simulink library "Loudness"  (R2022b)
settings: Solver=VariableStepAuto  StartTime=0.0  StopTime=10.0  RelTol=1e-3
InitFcn:
  | Loudness_init;
values from neighbouring files (symbols this model uses):
  COMP = struct('zipCoef', COMP_zipCoef,      'LoudBPFNum', COMPBASS_Num, 'LoudBPFDenom', COMPBASS_Denom,      'LoudLPFNum', COMPMID_Num, 'LoudLPFDenom', COMPMID_Denom,      'LoudBPFFreq',COMPBASS_Fc,'LoudBPFQ',COMPBASS_Q,      'LoudLPFFreq',COMPMID_Fc,'LoudLPFQ',COMPMID_Q)    [Loudness_init.m]
undefined symbols (not defined in the file or in its folder): dfilt, LOUD_BASS_0DB_SCALE, LOUD_BASS_D1, LOUD_BASS_D2, sys_defs
libraries: TuneVar x38, RTC x16, dspobslib x5
(part 1 of 2)
settings Model: Creator=jb10849  LastModifiedBy=kl13806
settings SolverCC: AlgebraicLoopSolver=TrustRegion
settings DebuggingCC: UnconnectedInputMsg=warning  UnconnectedOutputMsg=warning  UnconnectedLineMsg=warning  SFMachineParentedDataDiag=warning  ArithmeticOperatorsInVariantConditions=warning
settings ModelReferenceCC: EnableRefExpFcnMdlSchedulingChecks=on
settings SFSimCC: SimUseLocalCustomCode=off  CustomCodeUndefinedFunction=UseInterfaceOnly
settings RTWCC: RTWUseLocalCustomCode=off  DLArmComputeVersion=19.05
settings CodeAppCC: StateflowObjectComments=on

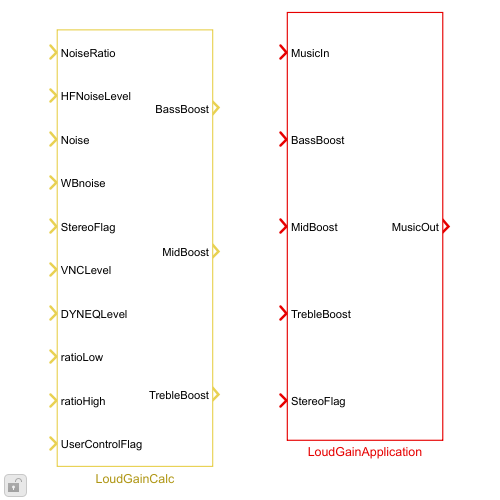
[thumbnail: Simulink's stored preview of the top-level diagram]
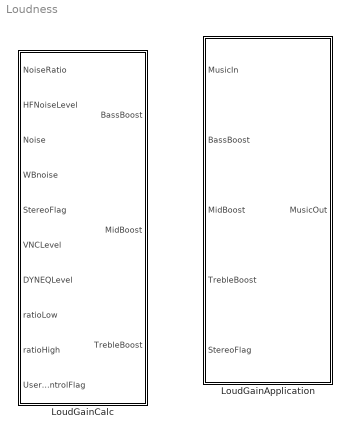
== system Loudness ==
  LoudGainApplication : Subsystem  mask(Loudness Gain Application){}
      mask help: Loudness gain application for Audio Pilot.
  LoudGainCalc : Subsystem  mask(Loudness Gain Calculation){}
      mask help: Loudness gain calculation for Audio Pilot.

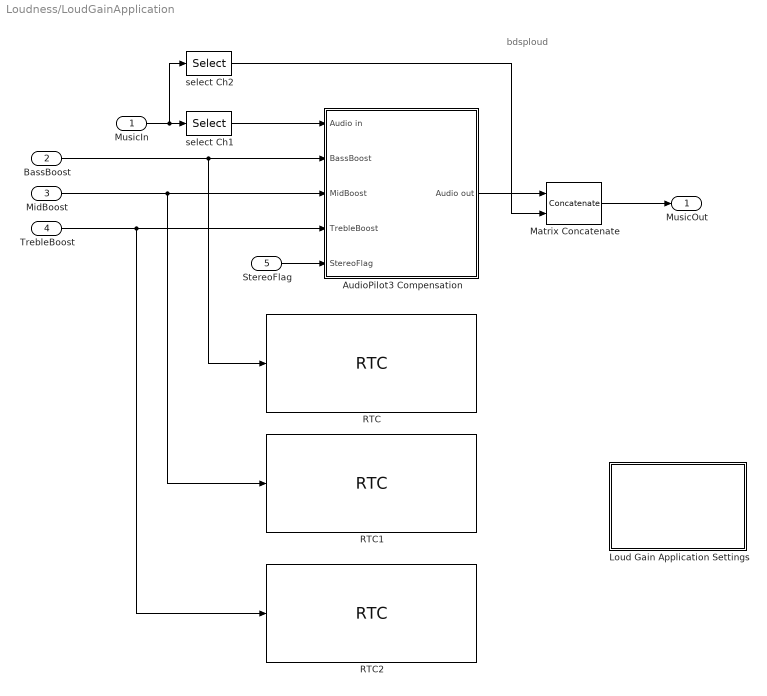
== system Loudness/LoudGainApplication ==
  note: bdsploud
  MusicIn : Inport
  BassBoost : Inport  Port=2
  MidBoost : Inport  Port=3
  TrebleBoost : Inport  Port=4
  StereoFlag : Inport  Port=5
  AudioPilot3 Compensation : Subsystem
  Loud Gain Application Settings : Subsystem
  Matrix Concatenate : Concatenate  Mode=Multidimensional array  ConcatenateDimension=2
  RTC : RTC/RTC  REQ_Priority=RTC_Mask.NormalPriority  RequestAtInit=off  EnableRequest=off  REQElemType1=single  REQElemWidth1=1  REQElemInitial1=[]  REQElemType2=uint32  REQElemWidth2=1  REQElemInitial2=[]  REQElemType3=uint32  REQElemWidth3=1  REQElemInitial3=[]  REQElemType4=uint32  REQElemWidth4=1  REQElemInitial4=[]  REQElemType5=uint32  REQElemWidth5=1  REQElemInitial5=[]  REQElemType6=uint32  REQElemWidth6=1  REQElemInitial6=[]  REQElemType7=uint32  REQElemWidth7=1  REQElemInitial7=[]  REQElemType8=uint32  REQElemWidth8=1  REQElemInitial8=[]  REQElemType9=uint32  REQElemWidth9=1  REQElemInitial9=[]  REQElemType10=uint32  REQElemWidth10=1  REQElemInitial10=[]  EnableResponse=on  EnableRSP_StatusIn=off  RSPElemName1=bassBoost  RSPElemType1=single  RSPElemWidth1=1  RSPElemType2=uint32  RSPElemWidth2=1  RSPElemType3=uint32  RSPElemWidth3=1  RSPElemType4=uint32  RSPElemWidth4=1  RSPElemType5=uint32  RSPElemWidth5=1  RSPElemType6=uint32  RSPElemWidth6=1  RSPElemType7=uint32  RSPElemWidth7=1  RSPElemType8=uint32  RSPElemWidth8=1  RSPElemType9=uint32  RSPElemWidth9=1  RSPElemType10=uint32  RSPElemWidth10=1  EnableNotification=off  EnableNTF_PrepTrig=off  NTFElemType1=uint32  NTFElemWidth1=1  NTFElemType2=uint32  NTFElemWidth2=1  NTFElemType3=uint32  NTFElemWidth3=1  NTFElemType4=uint32  NTFElemWidth4=1  NTFElemType5=uint32  NTFElemWidth5=1  NTFElemType6=uint32  NTFElemWidth6=1  NTFElemType7=uint32  NTFElemWidth7=1  NTFElemType8=uint32  NTFElemWidth8=1  NTFElemType9=uint32  NTFElemWidth9=1  NTFElemType10=uint32  NTFElemWidth10=1  MaskMessageName=getBassBoost
  RTC1 : RTC/RTC  REQ_Priority=RTC_Mask.NormalPriority  RequestAtInit=off  EnableRequest=off  REQElemType1=single  REQElemWidth1=1  REQElemInitial1=[]  REQElemType2=uint32  REQElemWidth2=1  REQElemInitial2=[]  REQElemType3=uint32  REQElemWidth3=1  REQElemInitial3=[]  REQElemType4=uint32  REQElemWidth4=1  REQElemInitial4=[]  REQElemType5=uint32  REQElemWidth5=1  REQElemInitial5=[]  REQElemType6=uint32  REQElemWidth6=1  REQElemInitial6=[]  REQElemType7=uint32  REQElemWidth7=1  REQElemInitial7=[]  REQElemType8=uint32  REQElemWidth8=1  REQElemInitial8=[]  REQElemType9=uint32  REQElemWidth9=1  REQElemInitial9=[]  REQElemType10=uint32  REQElemWidth10=1  REQElemInitial10=[]  EnableResponse=on  EnableRSP_StatusIn=off  RSPElemName1=midBoost  RSPElemType1=single  RSPElemWidth1=1  RSPElemType2=uint32  RSPElemWidth2=1  RSPElemType3=uint32  RSPElemWidth3=1  RSPElemType4=uint32  RSPElemWidth4=1  RSPElemType5=uint32  RSPElemWidth5=1  RSPElemType6=uint32  RSPElemWidth6=1  RSPElemType7=uint32  RSPElemWidth7=1  RSPElemType8=uint32  RSPElemWidth8=1  RSPElemType9=uint32  RSPElemWidth9=1  RSPElemType10=uint32  RSPElemWidth10=1  EnableNotification=off  EnableNTF_PrepTrig=off  NTFElemType1=uint32  NTFElemWidth1=1  NTFElemType2=uint32  NTFElemWidth2=1  NTFElemType3=uint32  NTFElemWidth3=1  NTFElemType4=uint32  NTFElemWidth4=1  NTFElemType5=uint32  NTFElemWidth5=1  NTFElemType6=uint32  NTFElemWidth6=1  NTFElemType7=uint32  NTFElemWidth7=1  NTFElemType8=uint32  NTFElemWidth8=1  NTFElemType9=uint32  NTFElemWidth9=1  NTFElemType10=uint32  NTFElemWidth10=1  MaskMessageName=getMidBoost
  RTC2 : RTC/RTC  REQ_Priority=RTC_Mask.NormalPriority  RequestAtInit=off  EnableRequest=off  REQElemType1=single  REQElemWidth1=1  REQElemInitial1=[]  REQElemType2=uint32  REQElemWidth2=1  REQElemInitial2=[]  REQElemType3=uint32  REQElemWidth3=1  REQElemInitial3=[]  REQElemType4=uint32  REQElemWidth4=1  REQElemInitial4=[]  REQElemType5=uint32  REQElemWidth5=1  REQElemInitial5=[]  REQElemType6=uint32  REQElemWidth6=1  REQElemInitial6=[]  REQElemType7=uint32  REQElemWidth7=1  REQElemInitial7=[]  REQElemType8=uint32  REQElemWidth8=1  REQElemInitial8=[]  REQElemType9=uint32  REQElemWidth9=1  REQElemInitial9=[]  REQElemType10=uint32  REQElemWidth10=1  REQElemInitial10=[]  EnableResponse=on  EnableRSP_StatusIn=off  RSPElemName1=trebleBoost  RSPElemType1=single  RSPElemWidth1=1  RSPElemType2=uint32  RSPElemWidth2=1  RSPElemType3=uint32  RSPElemWidth3=1  RSPElemType4=uint32  RSPElemWidth4=1  RSPElemType5=uint32  RSPElemWidth5=1  RSPElemType6=uint32  RSPElemWidth6=1  RSPElemType7=uint32  RSPElemWidth7=1  RSPElemType8=uint32  RSPElemWidth8=1  RSPElemType9=uint32  RSPElemWidth9=1  RSPElemType10=uint32  RSPElemWidth10=1  EnableNotification=off  EnableNTF_PrepTrig=off  NTFElemType1=uint32  NTFElemWidth1=1  NTFElemType2=uint32  NTFElemWidth2=1  NTFElemType3=uint32  NTFElemWidth3=1  NTFElemType4=uint32  NTFElemWidth4=1  NTFElemType5=uint32  NTFElemWidth5=1  NTFElemType6=uint32  NTFElemWidth6=1  NTFElemType7=uint32  NTFElemWidth7=1  NTFElemType8=uint32  NTFElemWidth8=1  NTFElemType9=uint32  NTFElemWidth9=1  NTFElemType10=uint32  NTFElemWidth10=1  MaskMessageName=getTrebleBoost
  select Ch1 : Selector  NumberOfDimensions=2  InputPortWidth=3  IndexOptions=Select all,Index vector (dialog)  Indices=[1 3],1:2  OutputSizes=1,1
  select Ch2 : Selector  NumberOfDimensions=2  InputPortWidth=3  IndexOptions=Select all,Index vector (dialog)  Indices=[1 3],3:6  OutputSizes=1,1
  MusicOut : Outport  VectorParamsAs1DForOutWhenUnconnected=off
  wires:
  MusicIn/1 -> select Ch2/1, select Ch1/1
  MidBoost/1 -> AudioPilot3 Compensation/3(MidBoost), RTC1/1
  TrebleBoost/1 -> AudioPilot3 Compensation/4(TrebleBoost), RTC2/1
  BassBoost/1 -> AudioPilot3 Compensation/2(BassBoost), RTC/1
  select Ch1/1 -> AudioPilot3 Compensation/1(Audio in)
  AudioPilot3 Compensation/1(Audio out) -> Matrix Concatenate/1
  Matrix Concatenate/1 -> MusicOut/1
  select Ch2/1 -> Matrix Concatenate/2
  StereoFlag/1 -> AudioPilot3 Compensation/5(StereoFlag)

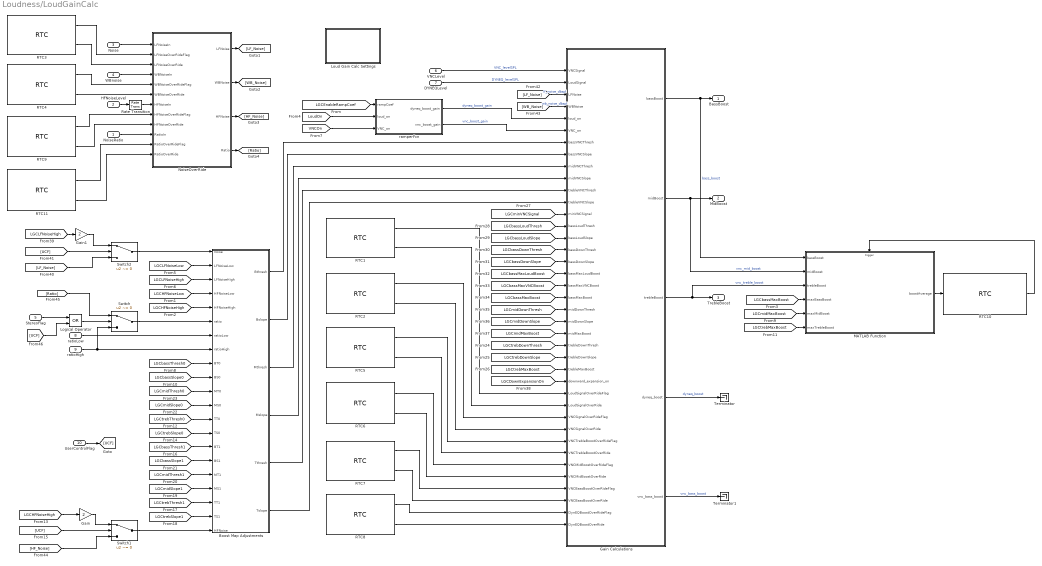
== system Loudness/LoudGainCalc ==
  NoiseRatio : Inport
  HFNoiseLevel : Inport  Port=2
  Noise : Inport  Port=3
  WBnoise : Inport  Port=4
  StereoFlag : Inport  Port=5
  VNCLevel : Inport  Port=6
  DYNEQLevel : Inport  Port=7
  ratioLow : Inport  Port=8
  ratioHigh : Inport  Port=9
  UserControlFlag : Inport  Port=10
  Boost Map Adjustments : MATLAB Function  TreatAsAtomicUnit=on
  Gain : Gain  Gain=2
  Gain Calculations : MATLAB Function  TreatAsAtomicUnit=on
  Gain1 : Gain  Gain=2
  Logical Operator : Logic  Operator=OR  AllPortsSameDT=off  OutDataTypeStr=boolean
  Loud Gain Calc Settings : Subsystem
  MATLAB Function : MATLAB Function  TreatAsAtomicUnit=on
  NoiseOverRide : MATLAB Function  TreatAsAtomicUnit=on
  RTC1 : RTC/RTC  REQ_Priority=RTC_Mask.NormalPriority  RequestAtInit=off  EnableRequest=off  REQElemName1=LoudSignalOverRideFlag  REQElemType1=uint32  REQElemWidth1=1  REQElemInitial1=[]  REQElemName2=LoudSignalOverRide  REQElemType2=single  REQElemWidth2=1  REQElemInitial2=[]  REQElemType3=uint32  REQElemWidth3=1  REQElemInitial3=[]  REQElemType4=uint32  REQElemWidth4=1  REQElemInitial4=[]  REQElemType5=uint32  REQElemWidth5=1  REQElemInitial5=[]  REQElemType6=uint32  REQElemWidth6=1  REQElemInitial6=[]  REQElemType7=uint32  REQElemWidth7=1  REQElemInitial7=[]  REQElemType8=uint32  REQElemWidth8=1  REQElemInitial8=[]  REQElemType9=uint32  REQElemWidth9=1  REQElemInitial9=[]  REQElemType10=uint32  REQElemWidth10=1  REQElemInitial10=[]  EnableResponse=off  EnableRSP_StatusIn=off  RSPElemType1=uint32  RSPElemWidth1=1  RSPElemType2=uint32  RSPElemWidth2=1  RSPElemType3=uint32  RSPElemWidth3=1  RSPElemType4=uint32  RSPElemWidth4=1  RSPElemType5=uint32  RSPElemWidth5=1  RSPElemType6=uint32  RSPElemWidth6=1  RSPElemType7=uint32  RSPElemWidth7=1  RSPElemType8=uint32  RSPElemWidth8=1  RSPElemType9=uint32  RSPElemWidth9=1  RSPElemType10=uint32  RSPElemWidth10=1  EnableNotification=off  EnableNTF_PrepTrig=off  NTFElemType1=uint32  NTFElemWidth1=1  NTFElemType2=uint32  NTFElemWidth2=1  NTFElemType3=uint32  NTFElemWidth3=1  NTFElemType4=uint32  NTFElemWidth4=1  NTFElemType5=uint32  NTFElemWidth5=1  NTFElemType6=uint32  NTFElemWidth6=1  NTFElemType7=uint32  NTFElemWidth7=1  NTFElemType8=uint32  NTFElemWidth8=1  NTFElemType9=uint32  NTFElemWidth9=1  NTFElemType10=uint32  NTFElemWidth10=1  MaskMessageName=setLoudSignalOverRide
  RTC10 : RTC/RTC  REQ_Priority=RTC_Mask.NormalPriority  RequestAtInit=off  EnableRequest=on  REQElemType1=uint32  REQElemWidth1=1  REQElemInitial1=[]  REQElemType2=uint32  REQElemWidth2=1  REQElemInitial2=[]  REQElemType3=uint32  REQElemWidth3=1  REQElemInitial3=[]  REQElemType4=uint32  REQElemWidth4=1  REQElemInitial4=[]  REQElemType5=uint32  REQElemWidth5=1  REQElemInitial5=[]  REQElemType6=uint32  REQElemWidth6=1  REQElemInitial6=[]  REQElemType7=uint32  REQElemWidth7=1  REQElemInitial7=[]  REQElemType8=uint32  REQElemWidth8=1  REQElemInitial8=[]  REQElemType9=uint32  REQElemWidth9=1  REQElemInitial9=[]  REQElemType10=uint32  REQElemWidth10=1  REQElemInitial10=[]  EnableResponse=on  EnableRSP_StatusIn=off  RSPElemName1=level  RSPElemType1=single  RSPElemWidth1=1  RSPElemType2=uint32  RSPElemWidth2=1  RSPElemType3=uint32  RSPElemWidth3=1  RSPElemType4=uint32  RSPElemWidth4=1  RSPElemType5=uint32  RSPElemWidth5=1  RSPElemType6=uint32  RSPElemWidth6=1  RSPElemType7=uint32  RSPElemWidth7=1  RSPElemType8=uint32  RSPElemWidth8=1  RSPElemType9=uint32  RSPElemWidth9=1  RSPElemType10=uint32  RSPElemWidth10=1  EnableNotification=off  EnableNTF_PrepTrig=off  NTFElemType1=uint32  NTFElemWidth1=1  NTFElemType2=uint32  NTFElemWidth2=1  NTFElemType3=uint32  NTFElemWidth3=1  NTFElemType4=uint32  NTFElemWidth4=1  NTFElemType5=uint32  NTFElemWidth5=1  NTFElemType6=uint32  NTFElemWidth6=1  NTFElemType7=uint32  NTFElemWidth7=1  NTFElemType8=uint32  NTFElemWidth8=1  NTFElemType9=uint32  NTFElemWidth9=1  NTFElemType10=uint32  NTFElemWidth10=1  MaskMessageName=getAverageAudioPilotBoostLevel
  RTC11 : RTC/RTC  REQ_Priority=RTC_Mask.NormalPriority  RequestAtInit=off  EnableRequest=off  REQElemName1=RatioOverRideFlag  REQElemType1=uint32  REQElemWidth1=1  REQElemInitial1=[]  REQElemName2=RatioOverRide  REQElemType2=single  REQElemWidth2=1  REQElemInitial2=[]  REQElemType3=uint32  REQElemWidth3=1  REQElemInitial3=[]  REQElemType4=uint32  REQElemWidth4=1  REQElemInitial4=[]  REQElemType5=uint32  REQElemWidth5=1  REQElemInitial5=[]  REQElemType6=uint32  REQElemWidth6=1  REQElemInitial6=[]  REQElemType7=uint32  REQElemWidth7=1  REQElemInitial7=[]  REQElemType8=uint32  REQElemWidth8=1  REQElemInitial8=[]  REQElemType9=uint32  REQElemWidth9=1  REQElemInitial9=[]  REQElemType10=uint32  REQElemWidth10=1  REQElemInitial10=[]  EnableResponse=off  EnableRSP_StatusIn=off  RSPElemType1=uint32  RSPElemWidth1=1  RSPElemType2=uint32  RSPElemWidth2=1  RSPElemType3=uint32  RSPElemWidth3=1  RSPElemType4=uint32  RSPElemWidth4=1  RSPElemType5=uint32  RSPElemWidth5=1  RSPElemType6=uint32  RSPElemWidth6=1  RSPElemType7=uint32  RSPElemWidth7=1  RSPElemType8=uint32  RSPElemWidth8=1  RSPElemType9=uint32  RSPElemWidth9=1  RSPElemType10=uint32  RSPElemWidth10=1  EnableNotification=off  EnableNTF_PrepTrig=off  NTFElemType1=uint32  NTFElemWidth1=1  NTFElemType2=uint32  NTFElemWidth2=1  NTFElemType3=uint32  NTFElemWidth3=1  NTFElemType4=uint32  NTFElemWidth4=1  NTFElemType5=uint32  NTFElemWidth5=1  NTFElemType6=uint32  NTFElemWidth6=1  NTFElemType7=uint32  NTFElemWidth7=1  NTFElemType8=uint32  NTFElemWidth8=1  NTFElemType9=uint32  NTFElemWidth9=1  NTFElemType10=uint32  NTFElemWidth10=1  MaskMessageName=setRatioOverRide
  RTC2 : RTC/RTC  REQ_Priority=RTC_Mask.NormalPriority  RequestAtInit=off  EnableRequest=off  REQElemName1=VNCSignalOverRideFlag  REQElemType1=uint32  REQElemWidth1=1  REQElemInitial1=[]  REQElemName2=VNCSignalOverRide  REQElemType2=single  REQElemWidth2=1  REQElemInitial2=[]  REQElemType3=uint32  REQElemWidth3=1  REQElemInitial3=[]  REQElemType4=uint32  REQElemWidth4=1  REQElemInitial4=[]  REQElemType5=uint32  REQElemWidth5=1  REQElemInitial5=[]  REQElemType6=uint32  REQElemWidth6=1  REQElemInitial6=[]  REQElemType7=uint32  REQElemWidth7=1  REQElemInitial7=[]  REQElemType8=uint32  REQElemWidth8=1  REQElemInitial8=[]  REQElemType9=uint32  REQElemWidth9=1  REQElemInitial9=[]  REQElemType10=uint32  REQElemWidth10=1  REQElemInitial10=[]  EnableResponse=off  EnableRSP_StatusIn=off  RSPElemType1=uint32  RSPElemWidth1=1  RSPElemType2=uint32  RSPElemWidth2=1  RSPElemType3=uint32  RSPElemWidth3=1  RSPElemType4=uint32  RSPElemWidth4=1  RSPElemType5=uint32  RSPElemWidth5=1  RSPElemType6=uint32  RSPElemWidth6=1  RSPElemType7=uint32  RSPElemWidth7=1  RSPElemType8=uint32  RSPElemWidth8=1  RSPElemType9=uint32  RSPElemWidth9=1  RSPElemType10=uint32  RSPElemWidth10=1  EnableNotification=off  EnableNTF_PrepTrig=off  NTFElemType1=uint32  NTFElemWidth1=1  NTFElemType2=uint32  NTFElemWidth2=1  NTFElemType3=uint32  NTFElemWidth3=1  NTFElemType4=uint32  NTFElemWidth4=1  NTFElemType5=uint32  NTFElemWidth5=1  NTFElemType6=uint32  NTFElemWidth6=1  NTFElemType7=uint32  NTFElemWidth7=1  NTFElemType8=uint32  NTFElemWidth8=1  NTFElemType9=uint32  NTFElemWidth9=1  NTFElemType10=uint32  NTFElemWidth10=1  MaskMessageName=setVNCSignalOverRide
  RTC3 : RTC/RTC  REQ_Priority=RTC_Mask.NormalPriority  RequestAtInit=off  EnableRequest=off  REQElemName1=LFNoiseOverRideFlag  REQElemType1=uint32  REQElemWidth1=1  REQElemInitial1=[]  REQElemName2=LFNoiseOverRide  REQElemType2=single  REQElemWidth2=1  REQElemInitial2=[]  REQElemType3=uint32  REQElemWidth3=1  REQElemInitial3=[]  REQElemType4=uint32  REQElemWidth4=1  REQElemInitial4=[]  REQElemType5=uint32  REQElemWidth5=1  REQElemInitial5=[]  REQElemType6=uint32  REQElemWidth6=1  REQElemInitial6=[]  REQElemType7=uint32  REQElemWidth7=1  REQElemInitial7=[]  REQElemType8=uint32  REQElemWidth8=1  REQElemInitial8=[]  REQElemType9=uint32  REQElemWidth9=1  REQElemInitial9=[]  REQElemType10=uint32  REQElemWidth10=1  REQElemInitial10=[]  EnableResponse=off  EnableRSP_StatusIn=off  RSPElemType1=uint32  RSPElemWidth1=1  RSPElemType2=uint32  RSPElemWidth2=1  RSPElemType3=uint32  RSPElemWidth3=1  RSPElemType4=uint32  RSPElemWidth4=1  RSPElemType5=uint32  RSPElemWidth5=1  RSPElemType6=uint32  RSPElemWidth6=1  RSPElemType7=uint32  RSPElemWidth7=1  RSPElemType8=uint32  RSPElemWidth8=1  RSPElemType9=uint32  RSPElemWidth9=1  RSPElemType10=uint32  RSPElemWidth10=1  EnableNotification=off  EnableNTF_PrepTrig=off  NTFElemType1=uint32  NTFElemWidth1=1  NTFElemType2=uint32  NTFElemWidth2=1  NTFElemType3=uint32  NTFElemWidth3=1  NTFElemType4=uint32  NTFElemWidth4=1  NTFElemType5=uint32  NTFElemWidth5=1  NTFElemType6=uint32  NTFElemWidth6=1  NTFElemType7=uint32  NTFElemWidth7=1  NTFElemType8=uint32  NTFElemWidth8=1  NTFElemType9=uint32  NTFElemWidth9=1  NTFElemType10=uint32  NTFElemWidth10=1  MaskMessageName=setLFNoiseOverRide
  RTC4 : RTC/RTC  REQ_Priority=RTC_Mask.NormalPriority  RequestAtInit=off  EnableRequest=off  REQElemName1=WBNoiseOverRideFlag  REQElemType1=uint32  REQElemWidth1=1  REQElemInitial1=[]  REQElemName2=WBNoiseOverRide  REQElemType2=single  REQElemWidth2=1  REQElemInitial2=[]  REQElemType3=uint32  REQElemWidth3=1  REQElemInitial3=[]  REQElemType4=uint32  REQElemWidth4=1  REQElemInitial4=[]  REQElemType5=uint32  REQElemWidth5=1  REQElemInitial5=[]  REQElemType6=uint32  REQElemWidth6=1  REQElemInitial6=[]  REQElemType7=uint32  REQElemWidth7=1  REQElemInitial7=[]  REQElemType8=uint32  REQElemWidth8=1  REQElemInitial8=[]  REQElemType9=uint32  REQElemWidth9=1  REQElemInitial9=[]  REQElemType10=uint32  REQElemWidth10=1  REQElemInitial10=[]  EnableResponse=off  EnableRSP_StatusIn=off  RSPElemType1=uint32  RSPElemWidth1=1  RSPElemType2=uint32  RSPElemWidth2=1  RSPElemType3=uint32  RSPElemWidth3=1  RSPElemType4=uint32  RSPElemWidth4=1  RSPElemType5=uint32  RSPElemWidth5=1  RSPElemType6=uint32  RSPElemWidth6=1  RSPElemType7=uint32  RSPElemWidth7=1  RSPElemType8=uint32  RSPElemWidth8=1  RSPElemType9=uint32  RSPElemWidth9=1  RSPElemType10=uint32  RSPElemWidth10=1  EnableNotification=off  EnableNTF_PrepTrig=off  NTFElemType1=uint32  NTFElemWidth1=1  NTFElemType2=uint32  NTFElemWidth2=1  NTFElemType3=uint32  NTFElemWidth3=1  NTFElemType4=uint32  NTFElemWidth4=1  NTFElemType5=uint32  NTFElemWidth5=1  NTFElemType6=uint32  NTFElemWidth6=1  NTFElemType7=uint32  NTFElemWidth7=1  NTFElemType8=uint32  NTFElemWidth8=1  NTFElemType9=uint32  NTFElemWidth9=1  NTFElemType10=uint32  NTFElemWidth10=1  MaskMessageName=setWBNoiseOverRide
  RTC5 : RTC/RTC  REQ_Priority=RTC_Mask.NormalPriority  RequestAtInit=off  EnableRequest=off  REQElemName1=VNCTrebleBoostOverRideFlag  REQElemType1=uint32  REQElemWidth1=1  REQElemInitial1=[]  REQElemName2=VNCTrebleBoostOverRide  REQElemType2=single  REQElemWidth2=1  REQElemInitial2=[]  REQElemType3=uint32  REQElemWidth3=1  REQElemInitial3=[]  REQElemType4=uint32  REQElemWidth4=1  REQElemInitial4=[]  REQElemType5=uint32  REQElemWidth5=1  REQElemInitial5=[]  REQElemType6=uint32  REQElemWidth6=1  REQElemInitial6=[]  REQElemType7=uint32  REQElemWidth7=1  REQElemInitial7=[]  REQElemType8=uint32  REQElemWidth8=1  REQElemInitial8=[]  REQElemType9=uint32  REQElemWidth9=1  REQElemInitial9=[]  REQElemType10=uint32  REQElemWidth10=1  REQElemInitial10=[]  EnableResponse=off  EnableRSP_StatusIn=off  RSPElemType1=uint32  RSPElemWidth1=1  RSPElemType2=uint32  RSPElemWidth2=1  RSPElemType3=uint32  RSPElemWidth3=1  RSPElemType4=uint32  RSPElemWidth4=1  RSPElemType5=uint32  RSPElemWidth5=1  RSPElemType6=uint32  RSPElemWidth6=1  RSPElemType7=uint32  RSPElemWidth7=1  RSPElemType8=uint32  RSPElemWidth8=1  RSPElemType9=uint32  RSPElemWidth9=1  RSPElemType10=uint32  RSPElemWidth10=1  EnableNotification=off  EnableNTF_PrepTrig=off  NTFElemType1=uint32  NTFElemWidth1=1  NTFElemType2=uint32  NTFElemWidth2=1  NTFElemType3=uint32  NTFElemWidth3=1  NTFElemType4=uint32  NTFElemWidth4=1  NTFElemType5=uint32  NTFElemWidth5=1  NTFElemType6=uint32  NTFElemWidth6=1  NTFElemType7=uint32  NTFElemWidth7=1  NTFElemType8=uint32  NTFElemWidth8=1  NTFElemType9=uint32  NTFElemWidth9=1  NTFElemType10=uint32  NTFElemWidth10=1  MaskMessageName=setVNCTrebleBoostOverRide
  RTC6 : RTC/RTC  REQ_Priority=RTC_Mask.NormalPriority  RequestAtInit=off  EnableRequest=off  REQElemName1=VNCMidBoostOverRideFlag  REQElemType1=uint32  REQElemWidth1=1  REQElemInitial1=[]  REQElemName2=VNCMidBoostOverRide  REQElemType2=single  REQElemWidth2=1  REQElemInitial2=[]  REQElemType3=uint32  REQElemWidth3=1  REQElemInitial3=[]  REQElemType4=uint32  REQElemWidth4=1  REQElemInitial4=[]  REQElemType5=uint32  REQElemWidth5=1  REQElemInitial5=[]  REQElemType6=uint32  REQElemWidth6=1  REQElemInitial6=[]  REQElemType7=uint32  REQElemWidth7=1  REQElemInitial7=[]  REQElemType8=uint32  REQElemWidth8=1  REQElemInitial8=[]  REQElemType9=uint32  REQElemWidth9=1  REQElemInitial9=[]  REQElemType10=uint32  REQElemWidth10=1  REQElemInitial10=[]  EnableResponse=off  EnableRSP_StatusIn=off  RSPElemType1=uint32  RSPElemWidth1=1  RSPElemType2=uint32  RSPElemWidth2=1  RSPElemType3=uint32  RSPElemWidth3=1  RSPElemType4=uint32  RSPElemWidth4=1  RSPElemType5=uint32  RSPElemWidth5=1  RSPElemType6=uint32  RSPElemWidth6=1  RSPElemType7=uint32  RSPElemWidth7=1  RSPElemType8=uint32  RSPElemWidth8=1  RSPElemType9=uint32  RSPElemWidth9=1  RSPElemType10=uint32  RSPElemWidth10=1  EnableNotification=off  EnableNTF_PrepTrig=off  NTFElemType1=uint32  NTFElemWidth1=1  NTFElemType2=uint32  NTFElemWidth2=1  NTFElemType3=uint32  NTFElemWidth3=1  NTFElemType4=uint32  NTFElemWidth4=1  NTFElemType5=uint32  NTFElemWidth5=1  NTFElemType6=uint32  NTFElemWidth6=1  NTFElemType7=uint32  NTFElemWidth7=1  NTFElemType8=uint32  NTFElemWidth8=1  NTFElemType9=uint32  NTFElemWidth9=1  NTFElemType10=uint32  NTFElemWidth10=1  MaskMessageName=setVNCMidBoostOverRide
  RTC7 : RTC/RTC  REQ_Priority=RTC_Mask.NormalPriority  RequestAtInit=off  EnableRequest=off  REQElemName1=VNCBassBoostOverRideFlag  REQElemType1=uint32  REQElemWidth1=1  REQElemInitial1=[]  REQElemName2=VNCBassBoostOverRide  REQElemType2=single  REQElemWidth2=1  REQElemInitial2=[]  REQElemType3=uint32  REQElemWidth3=1  REQElemInitial3=[]  REQElemType4=uint32  REQElemWidth4=1  REQElemInitial4=[]  REQElemType5=uint32  REQElemWidth5=1  REQElemInitial5=[]  REQElemType6=uint32  REQElemWidth6=1  REQElemInitial6=[]  REQElemType7=uint32  REQElemWidth7=1  REQElemInitial7=[]  REQElemType8=uint32  REQElemWidth8=1  REQElemInitial8=[]  REQElemType9=uint32  REQElemWidth9=1  REQElemInitial9=[]  REQElemType10=uint32  REQElemWidth10=1  REQElemInitial10=[]  EnableResponse=off  EnableRSP_StatusIn=off  RSPElemType1=uint32  RSPElemWidth1=1  RSPElemType2=uint32  RSPElemWidth2=1  RSPElemType3=uint32  RSPElemWidth3=1  RSPElemType4=uint32  RSPElemWidth4=1  RSPElemType5=uint32  RSPElemWidth5=1  RSPElemType6=uint32  RSPElemWidth6=1  RSPElemType7=uint32  RSPElemWidth7=1  RSPElemType8=uint32  RSPElemWidth8=1  RSPElemType9=uint32  RSPElemWidth9=1  RSPElemType10=uint32  RSPElemWidth10=1  EnableNotification=off  EnableNTF_PrepTrig=off  NTFElemType1=uint32  NTFElemWidth1=1  NTFElemType2=uint32  NTFElemWidth2=1  NTFElemType3=uint32  NTFElemWidth3=1  NTFElemType4=uint32  NTFElemWidth4=1  NTFElemType5=uint32  NTFElemWidth5=1  NTFElemType6=uint32  NTFElemWidth6=1  NTFElemType7=uint32  NTFElemWidth7=1  NTFElemType8=uint32  NTFElemWidth8=1  NTFElemType9=uint32  NTFElemWidth9=1  NTFElemType10=uint32  NTFElemWidth10=1  MaskMessageName=setVNCBassBoostOverRide
  RTC8 : RTC/RTC  REQ_Priority=RTC_Mask.NormalPriority  RequestAtInit=off  EnableRequest=off  REQElemName1=DynEQBoostOverRideFlag  REQElemType1=uint32  REQElemWidth1=1  REQElemInitial1=[]  REQElemName2=DynEQBoostOverRide  REQElemType2=single  REQElemWidth2=1  REQElemInitial2=[]  REQElemType3=uint32  REQElemWidth3=1  REQElemInitial3=[]  REQElemType4=uint32  REQElemWidth4=1  REQElemInitial4=[]  REQElemType5=uint32  REQElemWidth5=1  REQElemInitial5=[]  REQElemType6=uint32  REQElemWidth6=1  REQElemInitial6=[]  REQElemType7=uint32  REQElemWidth7=1  REQElemInitial7=[]  REQElemType8=uint32  REQElemWidth8=1  REQElemInitial8=[]  REQElemType9=uint32  REQElemWidth9=1  REQElemInitial9=[]  REQElemType10=uint32  REQElemWidth10=1  REQElemInitial10=[]  EnableResponse=off  EnableRSP_StatusIn=off  RSPElemType1=uint32  RSPElemWidth1=1  RSPElemType2=uint32  RSPElemWidth2=1  RSPElemType3=uint32  RSPElemWidth3=1  RSPElemType4=uint32  RSPElemWidth4=1  RSPElemType5=uint32  RSPElemWidth5=1  RSPElemType6=uint32  RSPElemWidth6=1  RSPElemType7=uint32  RSPElemWidth7=1  RSPElemType8=uint32  RSPElemWidth8=1  RSPElemType9=uint32  RSPElemWidth9=1  RSPElemType10=uint32  RSPElemWidth10=1  EnableNotification=off  EnableNTF_PrepTrig=off  NTFElemType1=uint32  NTFElemWidth1=1  NTFElemType2=uint32  NTFElemWidth2=1  NTFElemType3=uint32  NTFElemWidth3=1  NTFElemType4=uint32  NTFElemWidth4=1  NTFElemType5=uint32  NTFElemWidth5=1  NTFElemType6=uint32  NTFElemWidth6=1  NTFElemType7=uint32  NTFElemWidth7=1  NTFElemType8=uint32  NTFElemWidth8=1  NTFElemType9=uint32  NTFElemWidth9=1  NTFElemType10=uint32  NTFElemWidth10=1  MaskMessageName=setDynEQBoostOverRide
  RTC9 : RTC/RTC  REQ_Priority=RTC_Mask.NormalPriority  RequestAtInit=off  EnableRequest=off  REQElemName1=HFNoiseOverRideFlag  REQElemType1=uint32  REQElemWidth1=1  REQElemInitial1=[]  REQElemName2=HFNoiseOverRide  REQElemType2=single  REQElemWidth2=1  REQElemInitial2=[]  REQElemType3=uint32  REQElemWidth3=1  REQElemInitial3=[]  REQElemType4=uint32  REQElemWidth4=1  REQElemInitial4=[]  REQElemType5=uint32  REQElemWidth5=1  REQElemInitial5=[]  REQElemType6=uint32  REQElemWidth6=1  REQElemInitial6=[]  REQElemType7=uint32  REQElemWidth7=1  REQElemInitial7=[]  REQElemType8=uint32  REQElemWidth8=1  REQElemInitial8=[]  REQElemType9=uint32  REQElemWidth9=1  REQElemInitial9=[]  REQElemType10=uint32  REQElemWidth10=1  REQElemInitial10=[]  EnableResponse=off  EnableRSP_StatusIn=off  RSPElemType1=uint32  RSPElemWidth1=1  RSPElemType2=uint32  RSPElemWidth2=1  RSPElemType3=uint32  RSPElemWidth3=1  RSPElemType4=uint32  RSPElemWidth4=1  RSPElemType5=uint32  RSPElemWidth5=1  RSPElemType6=uint32  RSPElemWidth6=1  RSPElemType7=uint32  RSPElemWidth7=1  RSPElemType8=uint32  RSPElemWidth8=1  RSPElemType9=uint32  RSPElemWidth9=1  RSPElemType10=uint32  RSPElemWidth10=1  EnableNotification=off  EnableNTF_PrepTrig=off  NTFElemType1=uint32  NTFElemWidth1=1  NTFElemType2=uint32  NTFElemWidth2=1  NTFElemType3=uint32  NTFElemWidth3=1  NTFElemType4=uint32  NTFElemWidth4=1  NTFElemType5=uint32  NTFElemWidth5=1  NTFElemType6=uint32  NTFElemWidth6=1  NTFElemType7=uint32  NTFElemWidth7=1  NTFElemType8=uint32  NTFElemWidth8=1  NTFElemType9=uint32  NTFElemWidth9=1  NTFElemType10=uint32  NTFElemWidth10=1  MaskMessageName=setHFNoiseOverRide
  Rate Transition : RateTransition
  Switch : Switch  Criteria=u2 ~= 0  Threshold=0.5  SaturateOnIntegerOverflow=off  InputSameDT=off
  Switch1 : Switch  Criteria=u2 ~= 0  Threshold=0.5  SaturateOnIntegerOverflow=off  InputSameDT=off
  Switch2 : Switch  Criteria=u2 ~= 0  Threshold=0.5  SaturateOnIntegerOverflow=off  InputSameDT=off
  Terminator : Terminator
  Terminator1 : Terminator
  ramperFcn : MATLAB Function  TreatAsAtomicUnit=on
  BassBoost : Outport  VectorParamsAs1DForOutWhenUnconnected=off
  MidBoost : Outport  Port=2  VectorParamsAs1DForOutWhenUnconnected=off
  TrebleBoost : Outport  Port=3  VectorParamsAs1DForOutWhenUnconnected=off
  wires:
  ratioLow/1 -> Boost Map Adjustments/7(ratioLow)
  ratioHigh/1 -> Boost Map Adjustments/8(ratioHigh), Switch/3
  [LGCtrebThresh1] -> Boost Map Adjustments/19(TT1)
  [LGCtrebSlope1] -> Boost Map Adjustments/20(TS1)
  StereoFlag/1 -> Logical Operator/1
  Switch/1 -> Boost Map Adjustments/6(ratio)
  NoiseRatio/1 -> NoiseOverRide/10(RatioIn)
  VNCLevel/1 -> Gain Calculations/1(VNCSignal)  "VNC_levelSPL"
  Boost Map Adjustments/3(Mthresh) -> Gain Calculations/9(midVNCThresh)
  Boost Map Adjustments/4(Mslope) -> Gain Calculations/10(midVNCSlope)
  Boost Map Adjustments/1(Bthresh) -> Gain Calculations/7(bassVNCThresh)
  Boost Map Adjustments/2(Bslope) -> Gain Calculations/8(bassVNCSlope)
  Boost Map Adjustments/5(Tthresh) -> Gain Calculations/11(trebleVNCThresh)
  Boost Map Adjustments/6(Tslope) -> Gain Calculations/12(trebleVNCSlope)
  [LGCmidThresh0] -> Boost Map Adjustments/11(MT0)
  [LGCbassThresh1] -> Boost Map Adjustments/15(BT1)
  [LGCbassSlope1] -> Boost Map Adjustments/16(BS1)
  [LGCmidThresh1] -> Boost Map Adjustments/17(MT1)
  [LGCmidSlope1] -> Boost Map Adjustments/18(MS1)
  [LGCmidSlope0] -> Boost Map Adjustments/12(MS0)
  [LGCLFNoiseLow] -> Boost Map Adjustments/2(LFNoiseLow)
  [LGCLFNoiseHigh] -> Boost Map Adjustments/3(LFNoiseHigh)
  [LGCbassThresh0] -> Boost Map Adjustments/9(BT0)
  [LGCbassSlope0] -> Boost Map Adjustments/10(BS0)
  [LGCtrebSlope0] -> Boost Map Adjustments/14(TS0)
  [LGCtrebThresh0] -> Boost Map Adjustments/13(TT0)
  [LGCminVNCSignal] -> Gain Calculations/13(minVNCSignal)
  [LGCbassLoudThresh] -> Gain Calculations/14(bassLoudThresh)
  [LGCbassLoudSlope] -> Gain Calculations/15(bassLoudSlope)
  [LGCbassDownThresh] -> Gain Calculations/16(bassDownThresh)
  [LGCbassDownSlope] -> Gain Calculations/17(bassDownSlope)
  [LGCbassMaxLoudBoost] -> Gain Calculations/18(bassMaxLoudBoost)
  [LGCbassMaxVNCBoost] -> Gain Calculations/19(bassMaxVNCBoost)
  [LGCbassMaxBoost] -> Gain Calculations/20(bassMaxBoost)
  [LGCmidDownThresh] -> Gain Calculations/21(midDownThresh)
  [LGCmidDownSlope] -> Gain Calculations/22(midDownSlope)
  [LGCmidMaxBoost] -> Gain Calculations/23(midMaxBoost)
  [LGCtrebDownThresh] -> Gain Calculations/24(trebleDownThresh)
  [LGCtrebDownSlope] -> Gain Calculations/25(trebleDownSlope)
  [LGCtrebMaxBoost] -> Gain Calculations/26(trebleMaxBoost)
  [LGCDownExpansionOn] -> Gain Calculations/27(downward_expansion_on)
  HFNoiseLevel/1 -> Rate Transition/1
  [WB_Noise] -> Gain Calculations/4(WBNoise)  "wb_noise_dbspl"
  DYNEQLevel/1 -> Gain Calculations/2(LoudSignal)  "DYNEQ_levelSPL"
  RTC5/1 -> Gain Calculations/32(VNCTrebleBoostOverRideFlag)
  RTC5/2 -> Gain Calculations/33(VNCTrebleBoostOverRide)
  RTC1/1 -> Gain Calculations/28(LoudSignalOverRideFlag)
  RTC2/1 -> Gain Calculations/30(VNCSignalOverRideFlag)
  RTC2/2 -> Gain Calculations/31(VNCSignalOverRide)
  RTC7/1 -> Gain Calculations/36(VNCBassBoostOverRideFlag)
  RTC7/2 -> Gain Calculations/37(VNCBassBoostOverRide)
  RTC1/2 -> Gain Calculations/29(LoudSignalOverRide)
  RTC8/1 -> Gain Calculations/38(DynEQBoostOverRideFlag)
  RTC8/2 -> Gain Calculations/39(DynEQBoostOverRide)
  [LGCHFNoiseLow] -> Boost Map Adjustments/4(HFNoiseLow)
  [LGCHFNoiseHigh] -> Boost Map Adjustments/5(HFNoiseHigh)
  Gain Calculations/2(midBoost) -> MidBoost/1, MATLAB Function/2(midBoost)  "vnc_mid_boost"
  Gain Calculations/1(bassBoost) -> MATLAB Function/1(bassBoost), BassBoost/1  "bass_boost"
  Gain Calculations/3(trebleBoost) -> MATLAB Function/3(trebleBoost), TrebleBoost/1  "vnc_treble_boost"
  [LGCbassMaxBoost] -> MATLAB Function/4(maxBassBoost)
  [LGCmidMaxBoost] -> MATLAB Function/5(maxMidBoost)
  [LGCtrebMaxBoost] -> MATLAB Function/6(maxTrebleBoost)
  MATLAB Function/1(boostAverage) -> RTC10/1
  RTC10/1 -> MATLAB Function/Trigger
  Gain Calculations/4(dyneq_boost) -> Terminator/1  "dyneq_boost"
  Gain Calculations/5(vnc_bass_boost) -> Terminator1/1  "vnc_bass_boost"
  ramperFcn/1(dyneq_boost_gain) -> Gain Calculations/5(loud_on)  "dyneq_boost_gain"
  ramperFcn/2(vnc_boost_gain) -> Gain Calculations/6(VNC_on)  "vnc_boost_gain"
  [LoudOn] -> ramperFcn/2(loud_on)
  [VNCOn] -> ramperFcn/3(VNC_on)
  [LGCEnableRampCoef] -> ramperFcn/1(rampCoef)
  [UCF] -> Switch1/2
  Switch1/1 -> Boost Map Adjustments/21(HFNoise)
  [LGCHFNoiseHigh] -> Gain/1
  Gain/1 -> Switch1/1
  UserControlFlag/1 -> [UCF]
  [UCF] -> Switch2/2
  [LGCLFNoiseHigh] -> Gain1/1
  Gain1/1 -> Switch2/1
  Switch2/1 -> Boost Map Adjustments/1(noise)
  [LF_Noise] -> Switch2/3
  [LF_Noise] -> Gain Calculations/3(LFNoise)  "lf_noise_dbspl"
  RTC6/1 -> Gain Calculations/34(VNCMidBoostOverRideFlag)
  RTC6/2 -> Gain Calculations/35(VNCMidBoostOverRide)
  Rate Transition/1 -> NoiseOverRide/7(HFNoiseIn)
  [HF_Noise] -> Switch1/3
  NoiseOverRide/3(HFNoise) -> [HF_Noise]
  NoiseOverRide/4(Ratio) -> [Ratio]
  [Ratio] -> Switch/1
  NoiseOverRide/2(WBNoise) -> [WB_Noise]
  NoiseOverRide/1(LFNoise) -> [LF_Noise]
  Noise/1 -> NoiseOverRide/1(LFNoiseIn)
  WBnoise/1 -> NoiseOverRide/4(WBNoiseIn)
  RTC3/1 -> NoiseOverRide/2(LFNoiseOverRideFlag)
  RTC3/2 -> NoiseOverRide/3(LFNoiseOverRide)
  RTC4/1 -> NoiseOverRide/5(WBNoiseOverRideFlag)
  RTC4/2 -> NoiseOverRide/6(WBNoiseOverRide)
  RTC9/1 -> NoiseOverRide/8(HFNoiseOverRideFlag)
  RTC9/2 -> NoiseOverRide/9(HFNoiseOverRide)
  RTC11/1 -> NoiseOverRide/11(RatioOverRideFlag)
  RTC11/2 -> NoiseOverRide/12(RatioOverRide)
  [UCF] -> Logical Operator/2
  Logical Operator/1 -> Switch/2

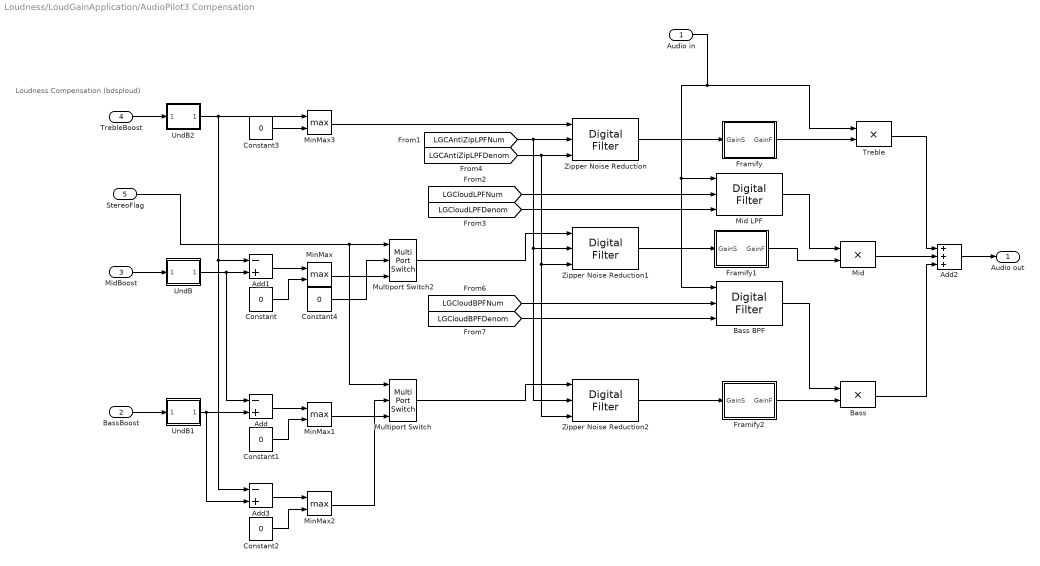
== system Loudness/LoudGainApplication/AudioPilot3 Compensation ==
  note: Loudness Compensation (bdsploud)
  Audio in : Inport
  BassBoost : Inport  Port=2
  MidBoost : Inport  Port=3
  TrebleBoost : Inport  Port=4
  StereoFlag : Inport  Port=5
  Add : Sum  Inputs=-+
  Add1 : Sum  Inputs=-+
  Add2 : Sum  Inputs=+++
  Add3 : Sum  Inputs=-+
  Bass : Product  InputSameDT=on  SaturateOnIntegerOverflow=on  OutDataTypeStr=Inherit: Same as first input
  Bass BPF : dspobslib/Digital Filter  TypePopup=IIR (poles & zeros)  IIRFiltStruct=Direct form II transposed  AllPoleFiltStruct=Direct form  FIRFiltStruct=Direct form  CoeffSource=Input port(s)  NumCoeffs=LOUD_BASS_0DB_SCALE*[1 0 -1]  DenCoeffs=[1 LOUD_BASS_D1 LOUD_BASS_D2]  BiQuadCoeffs=COMP.sosBass  LatticeCoeffs=[0.2 0.4]  denIgnore=on  FiltPerSampPopup=One filter per frame  IC=0  ICnum=0  ICden=0  roundingMode=Floor  overflowMode=off  ScaleValues=1  scaleValueFracLength=14  stageInFracLength=15  stageOutFracLength=15  FilterSource=Input port(s)  dfiltObjectName=dfilt.dffir([1 2 1])  InputProcessing=Inherited (this choice will be removed - see release notes)
  Constant{,1..4} (5 alike) : Constant  Value=0  OutDataTypeStr=single
  Framify : Subsystem  TreatAsAtomicUnit=on
  Framify1 : Subsystem  TreatAsAtomicUnit=on
  Framify2 : Subsystem  TreatAsAtomicUnit=on
  Mid : Product  InputSameDT=on  SaturateOnIntegerOverflow=on  OutDataTypeStr=Inherit: Same as first input
  Mid LPF : dspobslib/Digital Filter  TypePopup=IIR (poles & zeros)  IIRFiltStruct=Direct form II transposed  AllPoleFiltStruct=Direct form  FIRFiltStruct=Direct form  CoeffSource=Input port(s)  NumCoeffs=[1 2]  DenCoeffs=[1 0.1]  BiQuadCoeffs=COMP.sosMid  LatticeCoeffs=[0.2 0.4]  denIgnore=on  FiltPerSampPopup=One filter per frame  IC=0  ICnum=0  ICden=0  roundingMode=Floor  overflowMode=off  ScaleValues=1  scaleValueFracLength=14  stageInFracLength=15  stageOutFracLength=15  FilterSource=Input port(s)  dfiltObjectName=dfilt.dffir([1 2 1])  InputProcessing=Columns as channels (frame based)
  MinMax{,1..3} (4 alike) : MinMax  Function=max  Inputs=2
  Multiport Switch : MultiPortSwitch  DataPortOrder=Zero-based contiguous  Inputs=2  zeroidx=on  SaturateOnIntegerOverflow=off  InputSameDT=off
  Multiport Switch2 : MultiPortSwitch  DataPortOrder=Zero-based contiguous  Inputs=2  zeroidx=on  SaturateOnIntegerOverflow=off  InputSameDT=off
  Treble : Product  InputSameDT=on  SaturateOnIntegerOverflow=on  OutDataTypeStr=Inherit: Same as first input
  UndB : Subsystem  mask(dB Deconversion){}
      mask help: This block converts dB to amplitude.
  UndB1 : Subsystem  mask(dB Deconversion){}
      mask help: This block converts dB to amplitude.
  UndB2 : Subsystem  mask(dB Deconversion){}
      mask help: This block converts dB to amplitude.
  Zipper Noise Reduction : dspobslib/Digital Filter  TypePopup=IIR (poles & zeros)  IIRFiltStruct=Direct form II transposed  AllPoleFiltStruct=Direct form  FIRFiltStruct=Direct form  CoeffSource=Input port(s)  NumCoeffs=[1-COMP.zipCoef]  DenCoeffs=[1 -COMP.zipCoef]  BiQuadCoeffs=[1 0.3 0.4 1 0.1 0.2]  LatticeCoeffs=[0.2 0.4]  denIgnore=on  FiltPerSampPopup=One filter per frame  IC=0  ICnum=0  ICden=0  roundingMode=Floor  overflowMode=off  ScaleValues=1  scaleValueFracLength=14  stageInFracLength=15  stageOutFracLength=15  FilterSource=Input port(s)  dfiltObjectName=dfilt.dffir([1 2 1])  InputProcessing=Columns as channels (frame based)
  Zipper Noise Reduction1 : dspobslib/Digital Filter  TypePopup=IIR (poles & zeros)  IIRFiltStruct=Direct form II transposed  AllPoleFiltStruct=Direct form  FIRFiltStruct=Direct form  CoeffSource=Input port(s)  NumCoeffs=[1-COMP.zipCoef]  DenCoeffs=[1 -COMP.zipCoef]  BiQuadCoeffs=[1 0.3 0.4 1 0.1 0.2]  LatticeCoeffs=[0.2 0.4]  denIgnore=on  FiltPerSampPopup=One filter per frame  IC=0  ICnum=0  ICden=0  roundingMode=Floor  overflowMode=off  ScaleValues=1  scaleValueFracLength=14  stageInFracLength=15  stageOutFracLength=15  FilterSource=Input port(s)  dfiltObjectName=dfilt.dffir([1 2 1])  InputProcessing=Columns as channels (frame based)
  Zipper Noise Reduction2 : dspobslib/Digital Filter  TypePopup=IIR (poles & zeros)  IIRFiltStruct=Direct form II transposed  AllPoleFiltStruct=Direct form  FIRFiltStruct=Direct form  CoeffSource=Input port(s)  NumCoeffs=[1-COMP.zipCoef]  DenCoeffs=[1 -COMP.zipCoef]  BiQuadCoeffs=[1 0.3 0.4 1 0.1 0.2]  LatticeCoeffs=[0.2 0.4]  denIgnore=on  FiltPerSampPopup=One filter per frame  IC=0  ICnum=0  ICden=0  roundingMode=Floor  overflowMode=off  ScaleValues=1  scaleValueFracLength=14  stageInFracLength=15  stageOutFracLength=15  FilterSource=Input port(s)  dfiltObjectName=dfilt.dffir([1 2 1])  InputProcessing=Columns as channels (frame based)
  Audio out : Outport  VectorParamsAs1DForOutWhenUnconnected=off
  wires:
  Constant3/1 -> MinMax3/2
  TrebleBoost/1 -> UndB2/1(" ")
  MinMax3/1 -> Zipper Noise Reduction/1
  MinMax2/1 -> Multiport Switch/2
  MinMax1/1 -> Multiport Switch/3
  Multiport Switch/1 -> Zipper Noise Reduction2/1
  Constant2/1 -> MinMax2/2
  Add3/1 -> MinMax2/1
  Constant1/1 -> MinMax1/2
  Add/1 -> MinMax1/1
  Constant/1 -> MinMax/2
  Add1/1 -> MinMax/1
  UndB1/1("  ") -> Add3/2, Add/2
  Bass/1 -> Add2/3
  Bass BPF/1 -> Bass/1
  UndB2/1("  ") -> MinMax3/1, Add3/1, Add1/1
  Mid/1 -> Add2/2
  Treble/1 -> Add2/1
  UndB/1("  ") -> Add1/2, Add/1
  MidBoost/1 -> UndB/1(" ")
  BassBoost/1 -> UndB1/1(" ")
  Audio in/1 -> Mid LPF/1, Bass BPF/1, Treble/1
  MinMax/1 -> Multiport Switch2/3
  Constant4/1 -> Multiport Switch2/2
  Multiport Switch2/1 -> Zipper Noise Reduction1/1
  StereoFlag/1 -> Multiport Switch/1, Multiport Switch2/1
  Add2/1 -> Audio out/1
  Mid LPF/1 -> Mid/1
  Zipper Noise Reduction/1 -> Framify/1(GainS)
  [LGCloudLPFNum] -> Mid LPF/2
  [LGCloudLPFDenom] -> Mid LPF/3
  [LGCAntiZipLPFNum] -> Zipper Noise Reduction/2, Zipper Noise Reduction2/2, Zipper Noise Reduction1/2
  [LGCAntiZipLPFDenom] -> Zipper Noise Reduction/3, Zipper Noise Reduction2/3, Zipper Noise Reduction1/3
  Framify2/1(GainF) -> Bass/2
  Zipper Noise Reduction2/1 -> Framify2/1(GainS)
  Zipper Noise Reduction1/1 -> Framify1/1(GainS)
  Framify1/1(GainF) -> Mid/2
  Framify/1(GainF) -> Treble/2
  [LGCloudBPFNum] -> Bass BPF/2
  [LGCloudBPFDenom] -> Bass BPF/3

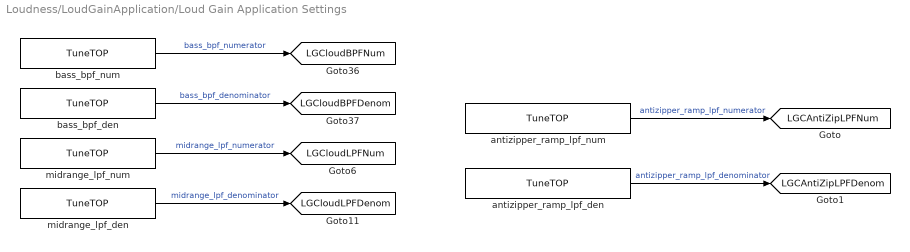
== system Loudness/LoudGainApplication/Loud Gain Application Settings ==
  antizipper_ramp_lpf_den : TuneVar/TuneTOP  TriggerInit=[-470 165 -305 195]  TopName=antizipper_ramp_lpf_denominator  TuneName=antizipper_ramp_lpf_denominator  DataType=Inherit: Same as input  PackageName=mode  BankNumber=0  TunabilityNumber=1  MinValue=[]  MaxValue=[]  UseSameName=on  MaskValue=single([1 -COMP.zipCoef])
  antizipper_ramp_lpf_num : TuneVar/TuneTOP  TriggerInit=[-470 100 -305 130]  TopName=antizipper_ramp_lpf_numerator  TuneName=antizipper_ramp_lpf_numerator  DataType=Inherit: Same as input  PackageName=mode  BankNumber=0  TunabilityNumber=1  MinValue=[]  MaxValue=[]  UseSameName=on  MaskValue=single(1-COMP.zipCoef)
  bass_bpf_den : TuneVar/TuneTOP  TriggerInit=[-915 85 -780 115]  TopName=bass_bpf_denominator  TuneName=bass_bpf_denominator  DataType=Inherit: Same as input  PackageName=mode  BankNumber=0  TunabilityNumber=1  MinValue=[]  MaxValue=[]  UseSameName=on  MaskValue=single(COMP.LoudBPFDenom)
  bass_bpf_num : TuneVar/TuneTOP  TriggerInit=[-915 35 -780 65]  TopName=bass_bpf_numerator  TuneName=bass_bpf_numerator  DataType=Inherit: Same as input  PackageName=mode  BankNumber=0  TunabilityNumber=1  MinValue=[]  MaxValue=[]  UseSameName=on  MaskValue=single(COMP.LoudBPFNum)
  midrange_lpf_den : TuneVar/TuneTOP  TriggerInit=[-915 185 -780 215]  TopName=midrange_lpf_denominator  TuneName=midrange_lpf_denominator  DataType=Inherit: Same as input  PackageName=mode  BankNumber=0  TunabilityNumber=1  MinValue=[]  MaxValue=[]  UseSameName=on  MaskValue=single(COMP.LoudLPFDenom)
  midrange_lpf_num : TuneVar/TuneTOP  TriggerInit=[-915 135 -780 165]  TopName=midrange_lpf_numerator  TuneName=midrange_lpf_numerator  DataType=Inherit: Same as input  PackageName=mode  BankNumber=0  TunabilityNumber=1  MinValue=[]  MaxValue=[]  UseSameName=on  MaskValue=single(COMP.LoudLPFNum)
  tag scope: LGCAntiZipLPFDenom=global, LGCAntiZipLPFNum=global, LGCloudBPFDenom=global, LGCloudBPFNum=global, LGCloudLPFDenom=global, LGCloudLPFNum=global
  wires:
  bass_bpf_num/1 -> [LGCloudBPFNum]  "bass_bpf_numerator"
  bass_bpf_den/1 -> [LGCloudBPFDenom]  "bass_bpf_denominator"
  antizipper_ramp_lpf_num/1 -> [LGCAntiZipLPFNum]  "antizipper_ramp_lpf_numerator"
  midrange_lpf_num/1 -> [LGCloudLPFNum]  "midrange_lpf_numerator"
  midrange_lpf_den/1 -> [LGCloudLPFDenom]  "midrange_lpf_denominator"
  antizipper_ramp_lpf_den/1 -> [LGCAntiZipLPFDenom]  "antizipper_ramp_lpf_denominator"
